simulink model "saturation"  (R2020a)
settings: Solver=VariableStepAuto  StartTime=0.0  StopTime=10.0  RelTol=1e-3
libraries: dspspect3 x1, simulink x1, dspsrcs4 x1
settings Model: Creator=XPS 15  LastModifiedBy=XPS 15

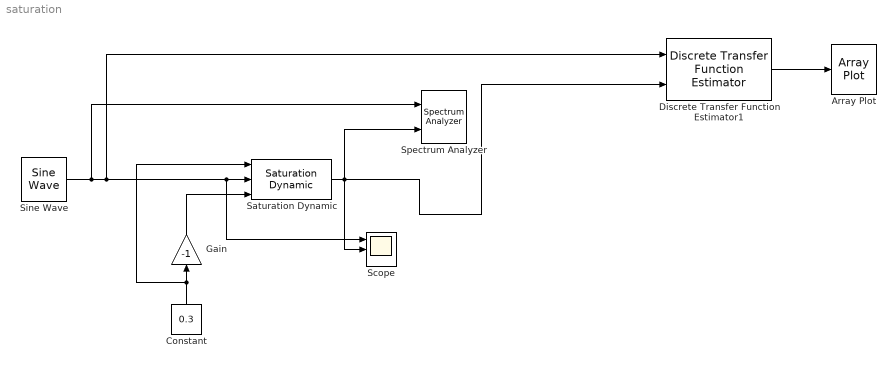
== system saturation ==
  Array Plot : ArrayPlot
  Constant : Constant  Value=0.3
  Discrete Transfer Function Estimator1 : dspspect3/Discrete Transfer Function Estimator  WindowMode=Specify on dialog  WindowLength=1024  Overlap=50  AveragingMethod=Running  ForgettingFactorPort=off  ForgettingFactor=0.9  SpectralAverages=100  FFTLengthSource=Auto  FFTLength=128  Window=Hann  SidelobeAttenuation=60  FrequencyRange=One-sided  OutputCoherence=off  SimulateUsing=Code generation
      settings: SourceProductBaseCode=DS
  Gain : Gain  Gain=-1
  Saturation Dynamic : simulink/Discontinuities/Saturation Dynamic  OutMin=[]  OutMax=[]  OutDataTypeStr=Inherit: Same as second input  OutDataType=fixdt(1, 16)  OutScaling=2^-10  DoSatur=off
  Scope : Scope  NumInputPorts=3
  Sine Wave : dspsrcs4/Sine Wave  Amplitude=1  Frequency=50  Phase=0  SampleMode=Discrete  OutComplex=Real  CompMethod=Trigonometric fcn  TableSize=Speed  SampleTime=1/10000  SamplesPerFrame=1  ResetState=Restart at time zero  OutputFrames=off  dataType=double  wordLen=16  udDataType=sfix(16)  fracBitsMode=Best precision  numFracBits=15  OutDataTypeStr=double  LastOutDataTypeStr=double
  Spectrum Analyzer : SpectrumAnalyzer  NumInputPorts=2
  wires:
  Gain/1 -> Saturation Dynamic/3
  Constant/1 -> Saturation Dynamic/1, Gain/1
  Sine Wave/1 -> Spectrum Analyzer/1, Discrete Transfer Function Estimator1/1, Scope/1, Saturation Dynamic/2
  Saturation Dynamic/1 -> Scope/2, Spectrum Analyzer/2, Discrete Transfer Function Estimator1/2
  Discrete Transfer Function Estimator1/1 -> Array Plot/1
